simulink model "P4_HardCode"  (R2020a)
settings: Solver=VariableStepAuto  StartTime=0.0  StopTime=20  RelTol=1e-3
model workspace (MAT data in the model file):
  A1 = 3
  A2 = 5
  R1 = 30
  R2 = 40
  g = 32.2
  h1_0 = 2
  h2_0 = 5
  rho = 1.94
undefined symbols (not defined in the file or in its folder): sgn
libraries: simulink x1
settings Model: Creator=Minghong.Xu19  LastModifiedBy=Minghong.Xu19

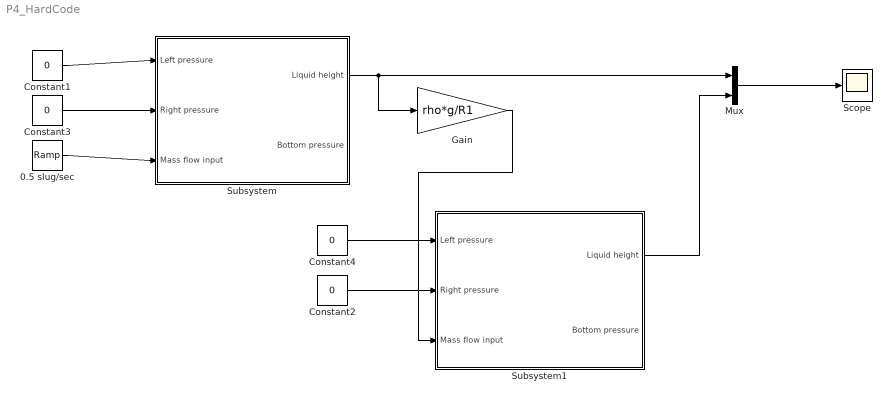
== system P4_HardCode ==
  0.5 slug/sec : simulink/Sources/Ramp  slope=0.5  start=0  InitialOutput=0
  Constant{1..4} (4 alike) : Constant  Value=0
  Gain : Gain  Gain=rho*g/R1
  Mux : Mux  Inputs=2
  Scope : Scope
  Subsystem : Subsystem
  Subsystem1 : Subsystem
  wires:
  Constant1/1 -> Subsystem/1(Left pressure)
  Constant2/1 -> Subsystem1/2(Right pressure)
  Subsystem/1(Liquid height) -> Mux/1, Gain/1
  Gain/1 -> Subsystem1/3(Mass flow input)
  Subsystem1/1(Liquid height) -> Mux/2
  Mux/1 -> Scope/1
  Constant3/1 -> Subsystem/2(Right pressure)
  Constant4/1 -> Subsystem1/1(Left pressure)
  0.5 slug/sec/1 -> Subsystem/3(Mass flow input)

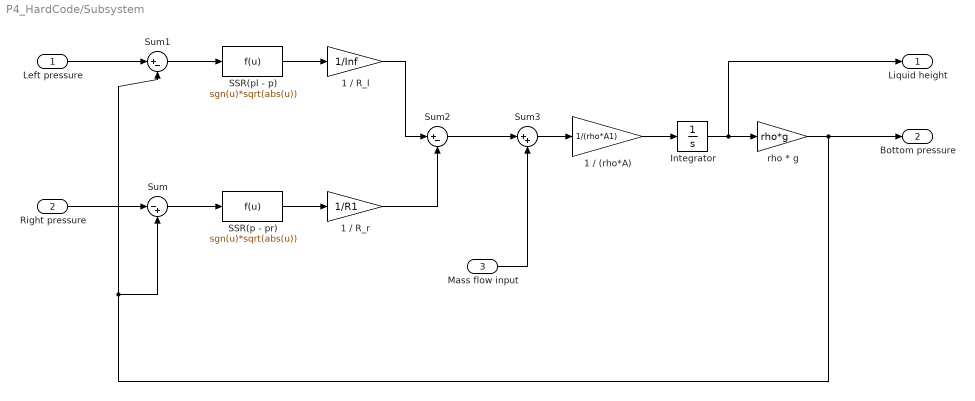
== system P4_HardCode/Subsystem ==
  Left pressure : Inport
  Right pressure : Inport  Port=2
  Mass flow input : Inport  Port=3
  1 / (rho*A) : Gain  Gain=1/(rho*A1)
  1 / R_l : Gain  Gain=1/Inf
  1 / R_r : Gain  Gain=1/R1
  Integrator : Integrator  InitialCondition=h1_0
  SSR(p - pr) : Fcn  Expr=sgn(u)*sqrt(abs(u))
  SSR(pl - p) : Fcn  Expr=sgn(u)*sqrt(abs(u))
  Sum : Sum  Inputs=|-+
  Sum1 : Sum  Inputs=|+-
  Sum2 : Sum  Inputs=|+-
  Sum3 : Sum  Inputs=|++
  rho * g : Gain  Gain=rho*g
  Liquid height : Outport
  Bottom pressure : Outport  Port=2
  wires:
  Sum2/1 -> Sum3/1
  SSR(p - pr)/1 -> 1 / R_r/1
  Sum1/1 -> SSR(pl - p)/1
  Right pressure/1 -> Sum/1
  Sum/1 -> SSR(p - pr)/1
  Integrator/1 -> Liquid height/1, rho * g/1
  1 / R_l/1 -> Sum2/1
  Sum3/1 -> 1 / (rho*A)/1
  SSR(pl - p)/1 -> 1 / R_l/1
  Mass flow input/1 -> Sum3/2
  1 / (rho*A)/1 -> Integrator/1
  Left pressure/1 -> Sum1/1
  rho * g/1 -> Bottom pressure/1, Sum/2, Sum1/2
  1 / R_r/1 -> Sum2/2

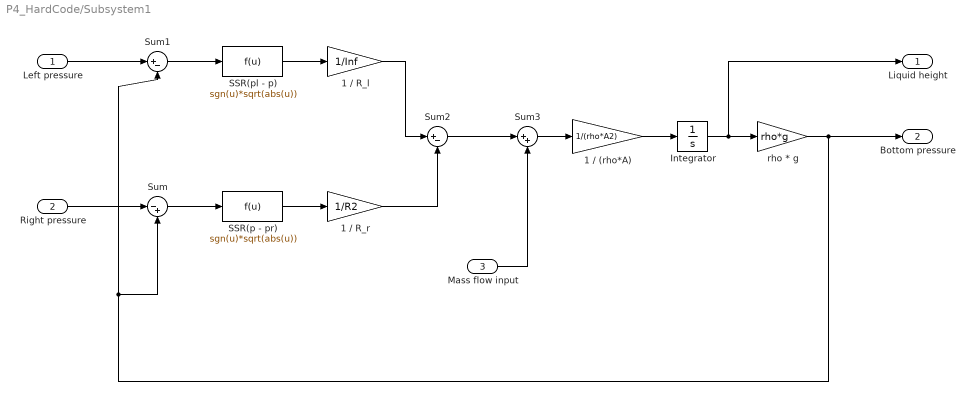
== system P4_HardCode/Subsystem1 ==
  Left pressure : Inport
  Right pressure : Inport  Port=2
  Mass flow input : Inport  Port=3
  1 / (rho*A) : Gain  Gain=1/(rho*A2)
  1 / R_l : Gain  Gain=1/Inf
  1 / R_r : Gain  Gain=1/R2
  Integrator : Integrator  InitialCondition=h2_0
  SSR(p - pr) : Fcn  Expr=sgn(u)*sqrt(abs(u))
  SSR(pl - p) : Fcn  Expr=sgn(u)*sqrt(abs(u))
  Sum : Sum  Inputs=|-+
  Sum1 : Sum  Inputs=|+-
  Sum2 : Sum  Inputs=|+-
  Sum3 : Sum  Inputs=|++
  rho * g : Gain  Gain=rho*g
  Liquid height : Outport
  Bottom pressure : Outport  Port=2
  wires:
  Sum2/1 -> Sum3/1
  SSR(p - pr)/1 -> 1 / R_r/1
  Sum1/1 -> SSR(pl - p)/1
  Right pressure/1 -> Sum/1
  Sum/1 -> SSR(p - pr)/1
  Integrator/1 -> Liquid height/1, rho * g/1
  1 / R_l/1 -> Sum2/1
  Sum3/1 -> 1 / (rho*A)/1
  SSR(pl - p)/1 -> 1 / R_l/1
  Mass flow input/1 -> Sum3/2
  1 / (rho*A)/1 -> Integrator/1
  Left pressure/1 -> Sum1/1
  rho * g/1 -> Bottom pressure/1, Sum/2, Sum1/2
  1 / R_r/1 -> Sum2/2
